simulink model "buck_converter"  (R2025a)
settings: Solver=VariableStepAuto  StartTime=0.0  StopTime=10.0  RelTol=1e-3
libraries: spsDCVoltageSourceLib x2, spsSeriesRLCBranchLib x2, spsDCMachineLib x1, spsDiodeLib x1, spsMosfetLib x1
settings Model: Creator=yiğit  LastModifiedBy=yiğit

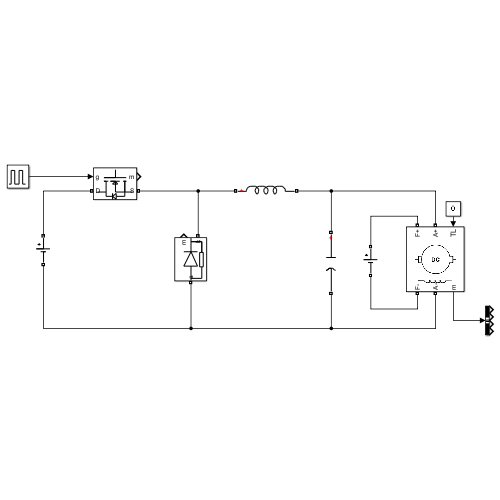
[thumbnail: Simulink's stored preview of the top-level diagram]
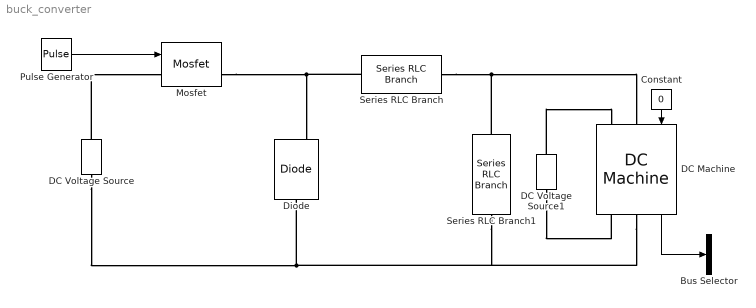
== system buck_converter ==
  Bus Selector : BusSelector  OutputSignals=Electrical torque Te (n m),Field current if (A),Armature current ia (A),Speed wm (rad/s)
  Constant : Constant  Value=0
  DC Machine : spsDCMachineLib/DC Machine  PresetModel=No  MechanicalLoad=Torque TL  FieldType=Wound  ShowDetailedParameters=on  MeasurementBus=off  RLa="[ 0.8  0.0125]"  RLf="[ 210  23]"  Laf=0  MachineConstant=Torque constant (N.m/A)  Ke=1.8  Kt=1.8  J=0.01  Bm=0.001  Tf=0  w0=1  Ifinit=1  TsPowergui=0  TsBlock=-1
  DC Voltage Source : spsDCVoltageSourceLib/DC Voltage Source  Amplitude=225  Measurements=None
  DC Voltage Source1 : spsDCVoltageSourceLib/DC Voltage Source  Amplitude=100  Measurements=None
  Diode : spsDiodeLib/Diode  Ron=0.001  Lon=0  Vf=0  IC=0  UseSnubber=0  Rs=1e6  Cs=1e-16  Measurements=on
  Mosfet : spsMosfetLib/Mosfet  Ron=0.1  Lon=0  Rd=0.01  Vfd=0  IC=0  Rs=1e5  Cs=inf  Measurements=on
  Pulse Generator : DiscretePulseGenerator  PulseType=Time based  Period=5e-5  PulseWidth=40
  Series RLC Branch : spsSeriesRLCBranchLib/Series RLC Branch  LConnTagsString=__new0  RConnTagsString=__new0  BranchType=L  Resistance=1  Inductance=500e-6  SetiL0=off  InitialCurrent=0  Capacitance=1e-6  Setx0=off  InitialVoltage=0  Measurements=None
  Series RLC Branch1 : spsSeriesRLCBranchLib/Series RLC Branch  LConnTagsString=__new0  RConnTagsString=__new0  BranchType=C  Resistance=1  Inductance=1e-3  SetiL0=off  InitialCurrent=0  Capacitance=220e-6  Setx0=off  InitialVoltage=0  Measurements=None
  wires:
  Constant/1 -> DC Machine/1
  Pulse Generator/1 -> Mosfet/1
  DC Machine/1 -> Bus Selector/1
  connections:
  DC Voltage Source/RConn1 -- Mosfet/LConn1
  Mosfet/RConn1 -- Series RLC Branch/LConn1 -- Diode/RConn1
  DC Voltage Source/LConn1 -- Series RLC Branch1/RConn1 -- DC Machine/RConn1 -- Diode/LConn1
  Series RLC Branch/RConn1 -- Series RLC Branch1/LConn1 -- DC Machine/LConn1
  DC Voltage Source1/RConn1 -- DC Machine/LConn2
  DC Voltage Source1/LConn1 -- DC Machine/RConn2
